simulink model "matrix"  (R2023b)
settings: Solver=VariableStepAuto  StartTime=0.0  StopTime=10.0  RelTol=1e-3
settings Model: Creator=NITRO  LastModifiedBy=NITRO

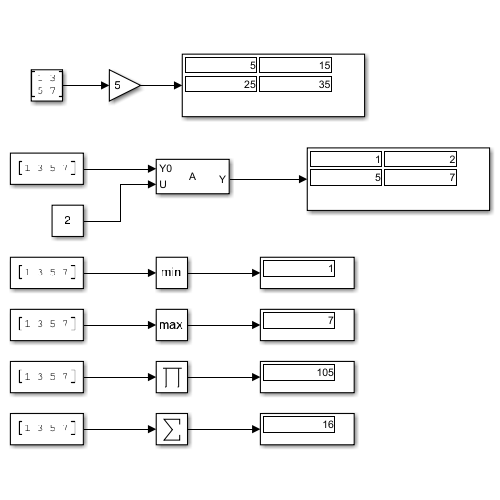
[thumbnail: Simulink's stored preview of the top-level diagram]
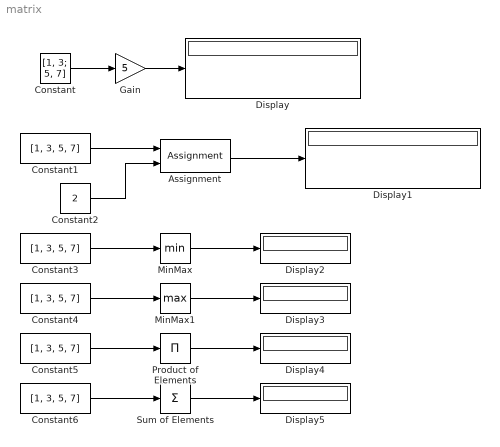
== system matrix ==
  Assignment : Assignment  DiagnosticForDimensions=Warning  IndexOptions=Index vector (dialog)  Indices=2  OutputSizes=1
  Constant : Constant  Value=[1, 3; 5, 7]
  Constant{1,3..6} (5 alike) : Constant  Value=[1, 3, 5, 7]
  Constant2 : Constant  Value=2
  Display{,1..5} (6 alike) : Display
  Gain : Gain  Gain=5
  MinMax : MinMax
  MinMax1 : MinMax  Function=max
  Product of Elements : Product  Inputs=*
  Sum of Elements : Sum  Inputs=+
  wires:
  Constant/1 -> Gain/1
  Gain/1 -> Display/1
  Constant1/1 -> Assignment/1
  Constant2/1 -> Assignment/2
  Assignment/1 -> Display1/1
  Constant3/1 -> MinMax/1
  MinMax/1 -> Display2/1
  Constant4/1 -> MinMax1/1
  MinMax1/1 -> Display3/1
  Constant5/1 -> Product of Elements/1
  Product of Elements/1 -> Display4/1
  Constant6/1 -> Sum of Elements/1
  Sum of Elements/1 -> Display5/1
